simulink model "final_block"  (R2021a)
settings: Solver=VariableStepAuto  StartTime=0.0  StopTime=0.05  RelTol=1e-3
undefined symbols (not defined in the file): K4, K5, R, T, T3, T4, T5, Tb, Tcd, Tg, Tl, Tm, Tt, Tv, Tw
settings Model: Creator=Souvik Datta  LastModifiedBy=Souvik Datta

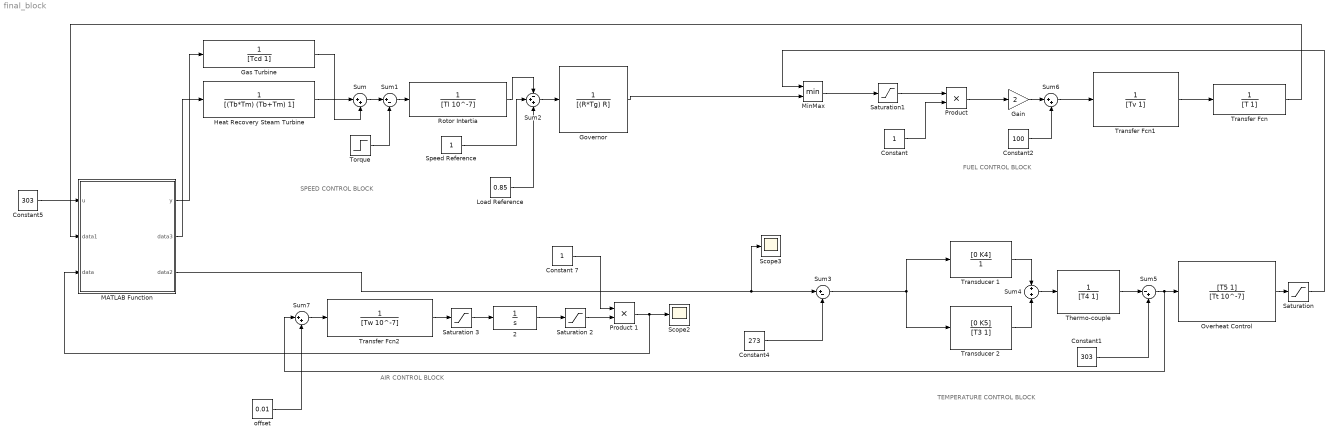
== system final_block ==
  note: TEMPERATURE CONTROL BLOCK
  note: SPEED CONTROL BLOCK
  note: AIR CONTROL BLOCK
  note: FUEL CONTROL BLOCK
  2 : TransferFcn  Denominator=[1 0]
  Constant : Constant
  Constant 7 : Constant
  Constant1 : Constant  Value=303
  Constant2 : Constant  Value=100
  Constant4 : Constant  Value=273
  Constant5 : Constant  Value=303
  Gain : Gain  Gain=2
  Gas Turbine : TransferFcn  Denominator=[Tcd 1]
  Governor : TransferFcn  Denominator=[(R*Tg) R]
  Heat Recovery Steam Turbine : TransferFcn  Denominator=[(Tb*Tm) (Tb+Tm) 1]
  Load Reference : Constant  Value=0.85
  MATLAB Function : MATLAB Function  TreatAsAtomicUnit=on
  MinMax : MinMax  Inputs=2
  Overheat Control : TransferFcn  Numerator=[T5 1]  Denominator=[Tt 10^-7]
  Product : Product
  Product 1 : Product
  Rotor Intertia : TransferFcn  Denominator=[Tl 10^-7]
  Saturation : Saturate  UpperLimit=350
  Saturation 2 : Saturate
  Saturation 3 : Saturate
  Saturation1 : Saturate
  Scope2 : Scope
  Scope3 : Scope
  Speed Reference : Constant
  Sum : Sum  Inputs=|++
  Sum1 : Sum  Inputs=|+-
  Sum2 : Sum  Inputs=-++
  Sum3 : Sum  Inputs=|+-
  Sum4 : Sum  Inputs=+|+
  Sum5 : Sum  Inputs=|-+
  Sum6 : Sum  Inputs=|++
  Sum7 : Sum  Inputs=|++
  Thermo-couple : TransferFcn  Denominator=[T4 1]
  Torque : Step  SampleTime=0
  Transducer 1 : TransferFcn  Numerator=[0 K4]  Denominator=[0 1]
  Transducer 2 : TransferFcn  Numerator=[0 K5]  Denominator=[T3 1]
  Transfer Fcn : TransferFcn  Denominator=[T 1]
  Transfer Fcn1 : TransferFcn  Denominator=[Tv 1]
  Transfer Fcn2 : TransferFcn  Denominator=[Tw 10^-7]
  offset : Constant  Value=0.01
  wires:
  Torque/1 -> Sum1/2
  Load Reference/1 -> Sum2/3
  Sum/1 -> Sum1/1
  Rotor Intertia/1 -> Sum2/1
  MATLAB Function/1(y) -> Gas Turbine/1
  Sum2/1 -> Governor/1
  Gas Turbine/1 -> Sum/2
  Sum1/1 -> Rotor Intertia/1
  Heat Recovery Steam Turbine/1 -> Sum/1
  Speed Reference/1 -> Sum2/2
  Overheat Control/1 -> Saturation/1
  MATLAB Function/3(data2) -> Scope3/1, Sum3/1
  Thermo-couple/1 -> Sum5/1
  Transducer 1/1 -> Sum4/1
  Constant1/1 -> Sum5/2
  Sum4/1 -> Thermo-couple/1
  Transducer 2/1 -> Sum4/2
  Sum3/1 -> Transducer 2/1, Transducer 1/1
  Saturation 3/1 -> 2/1
  Constant 7/1 -> Product 1/1
  Saturation 2/1 -> Product 1/2
  Sum7/1 -> Transfer Fcn2/1
  Sum5/1 -> Sum7/1, Overheat Control/1
  offset/1 -> Sum7/2
  Transfer Fcn2/1 -> Saturation 3/1
  2/1 -> Saturation 2/1
  Constant4/1 -> Sum3/2
  Sum6/1 -> Transfer Fcn1/1
  Transfer Fcn/1 -> MATLAB Function/2(data1)
  Constant/1 -> Product/2
  Governor/1 -> MinMax/2
  Saturation/1 -> MinMax/1
  Transfer Fcn1/1 -> Transfer Fcn/1
  Gain/1 -> Sum6/1
  Constant2/1 -> Sum6/2
  MinMax/1 -> Saturation1/1
  Product/1 -> Gain/1
  Saturation1/1 -> Product/1
  Constant5/1 -> MATLAB Function/1(u)
  Product 1/1 -> Scope2/1, MATLAB Function/3(data)
  MATLAB Function/2(data3) -> Heat Recovery Steam Turbine/1

== matlab function final_block/MATLAB Function ==
  data: u input; data1 input; y output; data3 output; data input; data2 output
function [y,data3, data2] = fcn(u, data1, data)

y = u;
